simulink model "BlockDiagramSimulink"  (R2025b)
settings: Solver=VariableStepAuto  StartTime=0.0  StopTime=10.0  RelTol=1e-3
settings Model: Creator=zahi  LastModifiedBy=zahi

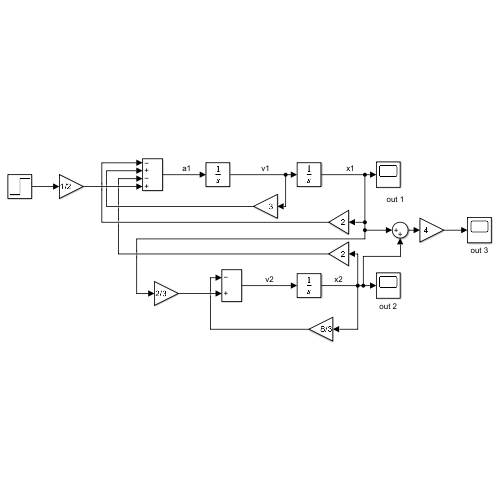
[thumbnail: Simulink's stored preview of the top-level diagram]
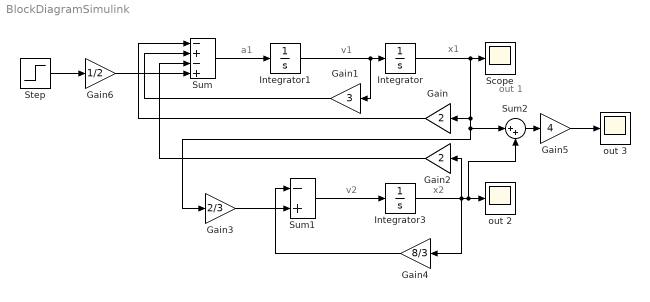
== system BlockDiagramSimulink ==
  note: a1
  note: v1
  note: x1
  note: out 1
  note: v2
  note: x2
  Gain : Gain  Gain=2
  Gain1 : Gain  Gain=3
  Gain2 : Gain  Gain=2
  Gain3 : Gain  Gain=2/3
  Gain4 : Gain  Gain=8/3
  Gain5 : Gain  Gain=4
  Gain6 : Gain  Gain=1/2
  Integrator : Integrator
  Integrator1 : Integrator
  Integrator3 : Integrator
  Scope : Scope
  Step : Step  SampleTime=0
  Sum : Sum  Inputs=-+-+
  Sum1 : Sum  Inputs=-+
  Sum2 : Sum  Inputs=|++
  out 2 : Scope
  out 3 : Scope
      settings: DataLoggingVariableName=ScopeData2
  wires:
  Integrator1/1 -> Gain1/1, Integrator/1
  Integrator/1 -> Sum2/1, Gain3/1, Gain/1, Scope/1
  Sum/1 -> Integrator1/1
  Gain/1 -> Sum/1
  Gain1/1 -> Sum/2
  Integrator3/1 -> Sum2/2, out 2/1, Gain4/1, Gain2/1
  Sum1/1 -> Integrator3/1
  Gain2/1 -> Sum/3
  Gain4/1 -> Sum1/1
  Gain3/1 -> Sum1/2
  Sum2/1 -> Gain5/1
  Gain5/1 -> out 3/1
  Gain6/1 -> Sum/4
  Step/1 -> Gain6/1
